simulink model "WECBench"  (R2025b)
settings: Solver=FixedStepAuto  StartTime=0.0  StopTime=inf  RelTol=1e-3
values from neighbouring files (symbols this model uses):
  CL = 13    [initWECBench.m]
  Damping = ExcelGains(:,2)    [initWECBench.m]
  driveKt = 23.6    [initWECBench.m]
  DUTKt = 8.51    [initWECBench.m]
  numPeriods = 10    [initWECBench.m]
  rampTime = 20    [initWECBench.m]
  sprocketPitchRadius = 0.0636651    [initWECBench.m]
  Stiffness = ExcelGains(:,1)    [initWECBench.m]
  Ts = 0.001    [initPendulum.m]    (also in initWECBench.m)
  wavePeriod = 6.00    (= 6)    [initWECBench.m]
libraries: slrealtimeethercatlib x38, slrealtimeloglib x13, dspfdesign x4, simulink x3, dspsrcs4 x2, dspsigops x1, slrealtimeptplib x1, slrealtimetgmanagement x1
settings Model: Creator=bbosma  LastModifiedBy=bosmab
settings SolverCC: ConcurrentTasks=on  PositivePriorityOrder=on
settings DataIOCC: ExternalInput=ds  LoadExternalInput=on
settings OptimizationCC: BlockReduction=off  OptimizeBlockIOStorage=off
settings DebuggingCC: TasksWithSamePriorityMsg=none
settings HardwareCC: ProdBitPerLong=64.0  ProdLongLongMode=on  ProdHWDeviceType=Intel->x86-64 (Linux 64)
settings RTWCC: SystemTargetFile=speedgoat.tlc  TemplateMakefile=slrealtime_default_tmf  RTWVerbose=off  Toolchain=Simulink Real-Time Toolchain  BuildConfiguration=Faster Runs  CodeExecutionProfiling=on  TargetLang=C++  Description=Speedgoat Real-Time Target Machine
settings SimulinkRealTimeTargetCC: SLRTFileLogMaxRuns=1.0  ExtModeMaxTrigDuration=10.0  ExtModeStaticAllocSize=1000000.0  ExtModeTransport=0.0  MultiwordLength=2048.0  DynamicStringBufferSize=256.0  PreserveMATLABNamespacesInGeneratedCode=on  SubcomponentCodeInterfacePackaging=Reusable function  MATLABClassNameForMDSCustomization=Simulink.SoftwareTarget.GRTCustomization  InstructionSetFMA=off  LogToMDFFile=off

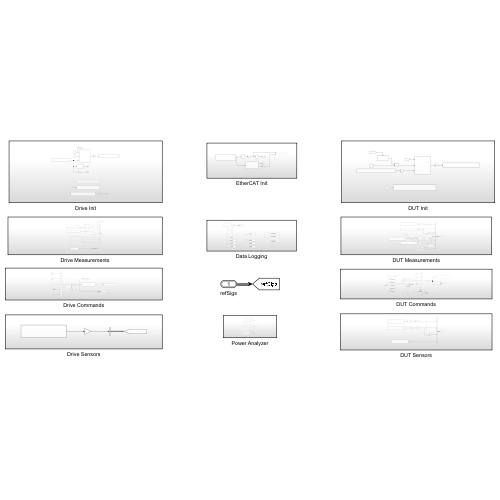
[thumbnail: Simulink's stored preview of the top-level diagram]
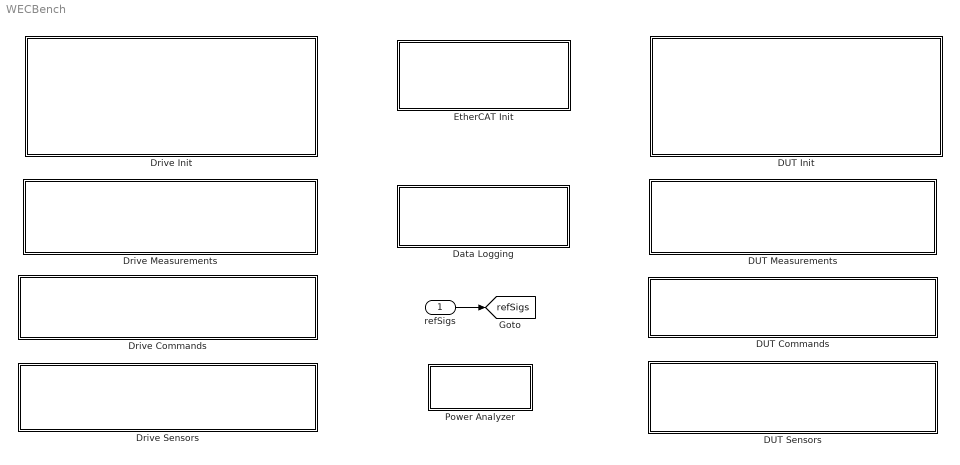
== system WECBench ==
  refSigs : Inport  OutDataTypeStr=Bus: refSigs
  DUT Commands : Subsystem
  DUT Init : Subsystem
  DUT Measurements : Subsystem
  DUT Sensors : Subsystem
  Data Logging : Subsystem
  Drive Commands : Subsystem
  Drive Init : Subsystem
  Drive Measurements : Subsystem
  Drive Sensors : Subsystem
  EtherCAT Init : Subsystem
  Power Analyzer : Subsystem
  tag scope: refSigs=global
  wires:
  refSigs/1 -> [refSigs]

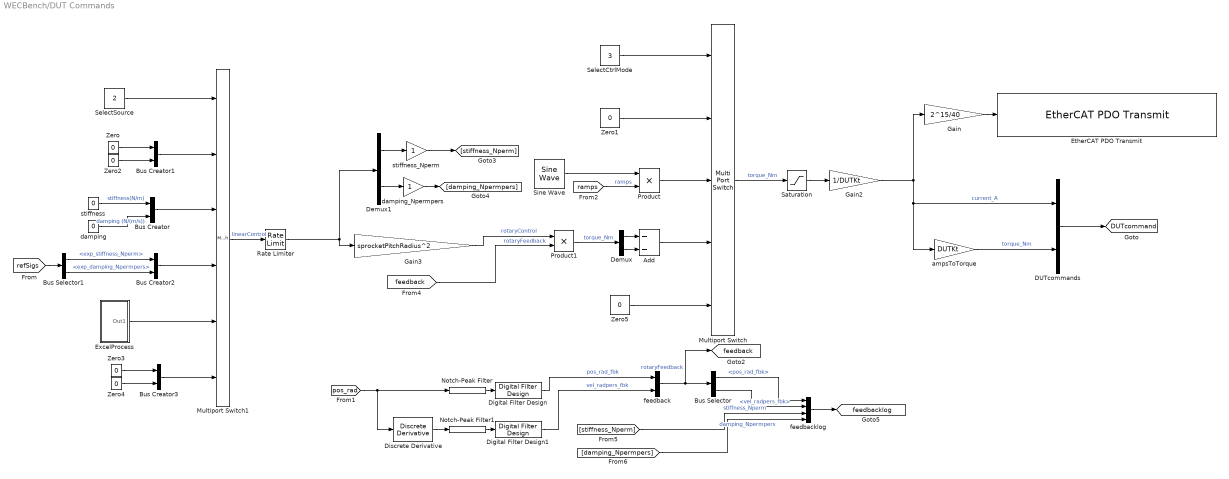
== system WECBench/DUT Commands ==
  Add : Sum  Inputs=--
  Bus Creator{,1..3} (4 alike) : BusCreator  Inputs=2
  Bus Selector : BusSelector  OutputSignals=pos_rad_fbk,vel_radpers_fbk
  Bus Selector1 : BusSelector  OutputSignals=exp_stiffness_Nperm,exp_damping_Npermpers
  DUTcommands : BusCreator  Inputs=2
  Demux : Demux  Outputs=2
  Demux1 : Demux  Outputs=2
  Digital Filter Design : dspfdesign/Digital Filter Design  mwdsp_browser_bugfix_var=off
  Digital Filter Design1 : dspfdesign/Digital Filter Design  mwdsp_browser_bugfix_var=off
  Discrete Derivative : simulink/Discrete/Discrete Derivative  gainval=1.0  ICPrevScaledInput=0.0  OutMin=[]  OutMax=[]  OutDataType=fixdt(1, 16)  OutScaling=2^-10  DoSatur=off
  EtherCAT PDO Transmit : slrealtimeethercatlib/EtherCAT PDO Transmit  Priority=3  sig_name=Drive 7 (AMC - DPE X2.1).PDO data to Slave.Target Current  sig_offset=656  sig_type=int16  type_size=16  sig_dim=1  device_id=0  sample_time=0.001000
  ExcelProcess : Subsystem
  Gain : Gain  Gain=2^15/40  OutDataTypeStr=int16
  Gain2 : Gain  Gain=1/DUTKt
  Gain3 : Gain  Gain=sprocketPitchRadius^2
  Multiport Switch : MultiPortSwitch  DataPortForDefault=Additional data port  SaturateOnIntegerOverflow=off  InputSameDT=off
  Multiport Switch1 : MultiPortSwitch  Inputs=4  DataPortForDefault=Additional data port  SaturateOnIntegerOverflow=off  InputSameDT=off
  Notch-Peak Filter : dspfdesign/Notch-Peak Filter  Specification=Bandwidth and center frequency  BandwidthPort=off  Bandwidth=10  QualityFactorPort=off  QualityFactor=5  CenterFrequencyPort=off  CenterFrequency=50  BandwidthCoefficientPort=off  BandwidthCoefficient=0.72654  CenterFrequencyCoefficientPort=off  CenterFrequencyCoefficient=0  Output=Notch  SampleRateMode=Specify on dialog  SampleRate=1/Ts  SimulateUsing=Code generation
  Notch-Peak Filter1 : dspfdesign/Notch-Peak Filter  Specification=Bandwidth and center frequency  BandwidthPort=off  Bandwidth=10  QualityFactorPort=off  QualityFactor=5  CenterFrequencyPort=off  CenterFrequency=50  BandwidthCoefficientPort=off  BandwidthCoefficient=0.72654  CenterFrequencyCoefficientPort=off  CenterFrequencyCoefficient=0  Output=Notch  SampleRateMode=Specify on dialog  SampleRate=1/Ts  SimulateUsing=Code generation
  Product : Product
  Product1 : Product
  Rate Limiter : RateLimiter  RisingSlewLimit=200  FallingSlewLimit=-200  SampleTimeMode=inherited
  Saturation : Saturate
  SelectCtrlMode : Constant  Value=3  OutDataTypeStr=double
  SelectSource : Constant  Value=2  OutDataTypeStr=double
  Sine Wave : dspsrcs4/Sine Wave  Amplitude=0.2*DUTKt  Frequency=1  Phase=0  SampleMode=Discrete  OutComplex=Real  CompMethod=Trigonometric fcn  TableSize=Speed  SampleTime=Ts  SamplesPerFrame=1  ResetState=Restart at time zero  OutputFrames=off  dataType=double  wordLen=16  udDataType=sfix(16)  fracBitsMode=Best precision  numFracBits=15  OutDataTypeStr=double  LastOutDataTypeStr=double
  Zero{,2..4} (4 alike) : Constant  Value=0  OutDataTypeStr=double
  Zero1 : Constant  Value=0  OutDataTypeStr=Inherit: Inherit via back propagation
  Zero5 : Constant  Value=0  OutDataTypeStr=Inherit: Inherit via back propagation
  ampsToTorque : Gain  Gain=DUTKt
  damping : Constant  Value=0  OutDataTypeStr=double
  damping_Npermpers : Gain
  feedback : BusCreator  Inputs=2
  feedbacklog : BusCreator  Inputs=4
  stiffness : Constant  Value=0  OutDataTypeStr=double
  stiffness_Nperm : Gain
  tag scope: DUTcommand=global, feedback=global, feedbacklog=global
  wires:
  Gain2/1 -> Gain/1, ampsToTorque/1, DUTcommands/1  "current_A"
  Gain/1 -> EtherCAT PDO Transmit/1
  ampsToTorque/1 -> DUTcommands/2  "torque_Nm"
  DUTcommands/1 -> [DUTcommand]
  SelectCtrlMode/1 -> Multiport Switch/1
  Zero1/1 -> Multiport Switch/2
  Multiport Switch/1 -> Saturation/1  "torque_Nm"
  [ramps] -> Product/2  "ramps"
  Sine Wave/1 -> Product/1
  Product/1 -> Multiport Switch/3
  Saturation/1 -> Gain2/1
  [pos_rad] -> Notch-Peak Filter/1, Discrete Derivative/1
  Discrete Derivative/1 -> Notch-Peak Filter1/1
  SelectSource/1 -> Multiport Switch1/1
  Digital Filter Design1/1 -> feedback/2  "vel_radpers_fbk"
  Digital Filter Design/1 -> feedback/1  "pos_rad_fbk"
  Bus Creator/1 -> Multiport Switch1/3
  [feedback] -> Product1/2  "rotaryFeedback"
  Multiport Switch1/1 -> Rate Limiter/1  "linearControl"
  Bus Creator1/1 -> Multiport Switch1/2
  Zero/1 -> Bus Creator1/1
  Demux/2 -> Add/2
  Demux/1 -> Add/1
  Add/1 -> Multiport Switch/4
  Zero2/1 -> Bus Creator1/2
  stiffness/1 -> Bus Creator/1  "stiffness(N/m)"
  damping/1 -> Bus Creator/2  "damping (N/(m/s))"
  feedback/1 -> Bus Selector/1, [feedback]  "rotaryFeedback"
  Product1/1 -> Demux/1  "torque_Nm"
  Gain3/1 -> Product1/1  "rotaryControl"
  [stiffness_Nperm] -> feedbacklog/3  "stiffness_Nperm"
  [damping_Npermpers] -> feedbacklog/4  "damping_Npermpers"
  feedbacklog/1 -> [feedbacklog]
  Bus Selector/2 -> feedbacklog/2  "<vel_radpers_fbk>"
  Bus Selector/1 -> feedbacklog/1  "<pos_rad_fbk>"
  Notch-Peak Filter/1 -> Digital Filter Design/1
  Notch-Peak Filter1/1 -> Digital Filter Design1/1
  [refSigs] -> Bus Selector1/1
  Bus Selector1/1 -> Bus Creator2/1  "<exp_stiffness_Nperm>"
  Bus Selector1/2 -> Bus Creator2/2  "<exp_damping_Npermpers>"
  Bus Creator2/1 -> Multiport Switch1/4
  Demux1/1 -> stiffness_Nperm/1
  Demux1/2 -> damping_Npermpers/1
  stiffness_Nperm/1 -> [stiffness_Nperm]
  damping_Npermpers/1 -> [damping_Npermpers]
  Rate Limiter/1 -> Gain3/1, Demux1/1
  Zero4/1 -> Bus Creator3/2
  Zero3/1 -> Bus Creator3/1
  Bus Creator3/1 -> Multiport Switch1/6
  Zero5/1 -> Multiport Switch/5
  ExcelProcess/1(Out1) -> Multiport Switch1/5

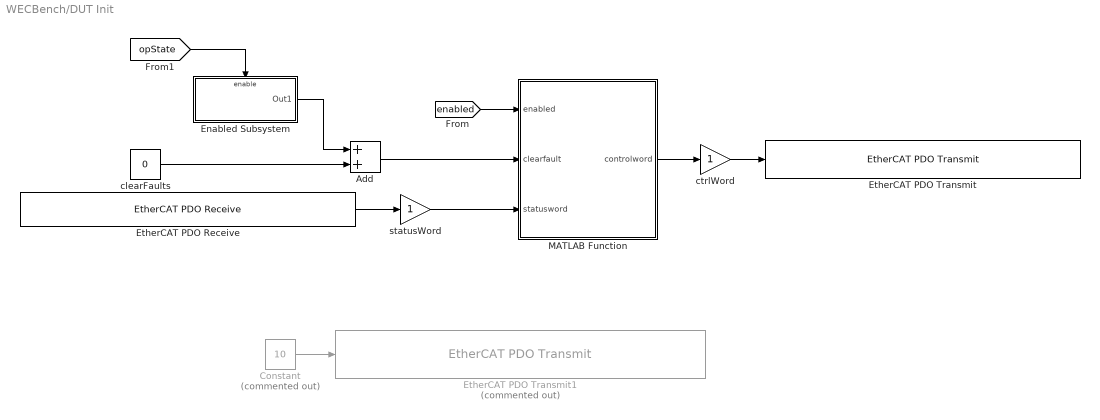
== system WECBench/DUT Init ==
  Add : Sum
  Constant : Constant  Commented=on  Value=10  OutDataTypeStr=int8
  Enabled Subsystem : Subsystem  TreatAsAtomicUnit=on
  EtherCAT PDO Receive : slrealtimeethercatlib/EtherCAT PDO Receive  Priority=2  sig_name=Drive 7 (AMC - DPE X2.1).PDO data from Slave.Status Word  sig_offset=576  sig_type=uint16  type_size=16  sig_dim=1  device_id=0  sample_time=0.001000
  EtherCAT PDO Transmit : slrealtimeethercatlib/EtherCAT PDO Transmit  Priority=3  sig_name=Drive 7 (AMC - DPE X2.1).PDO data to Slave.Control Word  sig_offset=576  sig_type=uint16  type_size=16  sig_dim=1  device_id=0  sample_time=0.001000
  EtherCAT PDO Transmit1 : slrealtimeethercatlib/EtherCAT PDO Transmit  Priority=3  Commented=on  sig_name=Drive 7 (AMC - DPE X2.1).PDO data to Slave.Modes Of Operation  sig_offset=688  sig_type=uint16  type_size=16  sig_dim=1  device_id=0  sample_time=0.001
  MATLAB Function : MATLAB Function  TreatAsAtomicUnit=on
  clearFaults : Constant  Value=0  OutDataTypeStr=Inherit: Inherit via back propagation
  ctrlWord : Gain  OutDataTypeStr=uint16
  statusWord : Gain  OutDataTypeStr=double
  wires:
  ctrlWord/1 -> EtherCAT PDO Transmit/1
  Constant/1 -> EtherCAT PDO Transmit1/1
  MATLAB Function/1(controlword) -> ctrlWord/1
  clearFaults/1 -> Add/2
  EtherCAT PDO Receive/1 -> statusWord/1
  [enabled] -> MATLAB Function/1(enabled)
  statusWord/1 -> MATLAB Function/3(statusword)
  [opState] -> Enabled Subsystem/Enable
  Enabled Subsystem/1(Out1) -> Add/1
  Add/1 -> MATLAB Function/2(clearfault)

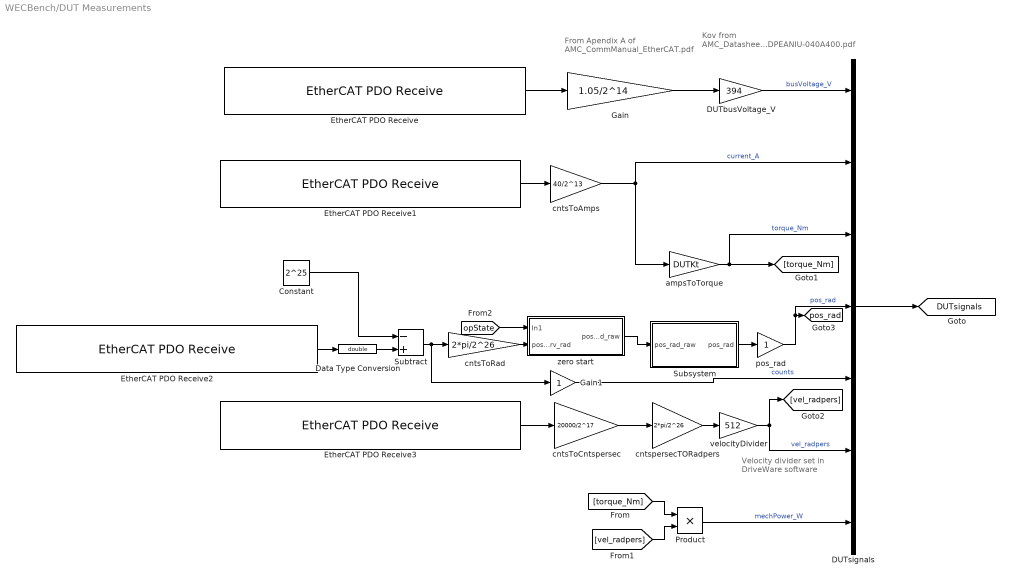
== system WECBench/DUT Measurements ==
  note: Velocity divider set in DriveWare software
  note: Kov from AMC_Datasheet_DPEANIU-040A400.pdf
  note: From Apendix A of AMC_CommManual_EtherCAT.pdf
  Constant : Constant  Value=2^25
  DUTbusVoltage_V : Gain  Gain=394
  DUTsignals : BusCreator  Inputs=7
  Data Type Conversion : DataTypeConversion  OutDataTypeStr=double  SaturateOnIntegerOverflow=off  RndMeth=Floor
  EtherCAT PDO Receive : slrealtimeethercatlib/EtherCAT PDO Receive  Priority=2  sig_name=Drive 7 (AMC - DPE X2.1).PDO data from Slave.DC Bus Voltage  sig_offset=688  sig_type=uint16  type_size=16  sig_dim=1  device_id=0  sample_time=0.001000
  EtherCAT PDO Receive1 : slrealtimeethercatlib/EtherCAT PDO Receive  Priority=2  sig_name=Drive 7 (AMC - DPE X2.1).PDO data from Slave.Actual Current  sig_offset=656  sig_type=int16  type_size=16  sig_dim=1  device_id=0  sample_time=0.001000
  EtherCAT PDO Receive2 : slrealtimeethercatlib/EtherCAT PDO Receive  Priority=2  sig_name=Drive 7 (AMC - DPE X2.1).PDO data from Slave.Actual position  sig_offset=592  sig_type=int32  type_size=32  sig_dim=1  device_id=0  sample_time=0.001000
  EtherCAT PDO Receive3 : slrealtimeethercatlib/EtherCAT PDO Receive  Priority=2  sig_name=Drive 7 (AMC - DPE X2.1).PDO data from Slave.Actual Velocity  sig_offset=624  sig_type=int32  type_size=32  sig_dim=1  device_id=0  sample_time=0.001000
  Gain : Gain  Gain=1.05/2^14  OutDataTypeStr=double
  Gain1 : Gain  OutDataTypeStr=double
  Product : Product
  Subsystem : Subsystem
  Subtract : Sum  Inputs=-+
  ampsToTorque : Gain  Gain=DUTKt
  cntsToAmps : Gain  Gain=40/2^13  OutDataTypeStr=double
  cntsToCntspersec : Gain  Gain=20000/2^17  OutDataTypeStr=double
  cntsToRad : Gain  Gain=2*pi/2^26  OutDataTypeStr=double
  cntspersecTORadpers : Gain  Gain=2*pi/2^26
  pos_rad : Gain
  velocityDivider : Gain  Gain=512
  zero start : Subsystem
  tag scope: DUTsignals=global, pos_rad=global
  wires:
  EtherCAT PDO Receive/1 -> Gain/1
  Gain/1 -> DUTbusVoltage_V/1
  DUTbusVoltage_V/1 -> DUTsignals/1  "busVoltage_V"
  DUTsignals/1 -> [DUTsignals]
  EtherCAT PDO Receive1/1 -> cntsToAmps/1
  cntsToAmps/1 -> ampsToTorque/1, DUTsignals/2  "current_A"
  ampsToTorque/1 -> DUTsignals/3, [torque_Nm]  "torque_Nm"
  Subtract/1 -> Gain1/1, cntsToRad/1
  pos_rad/1 -> [pos_rad], DUTsignals/4  "pos_rad"
  EtherCAT PDO Receive3/1 -> cntsToCntspersec/1
  cntsToCntspersec/1 -> cntspersecTORadpers/1
  cntspersecTORadpers/1 -> velocityDivider/1
  velocityDivider/1 -> [vel_radpers], DUTsignals/6  "vel_radpers"
  [torque_Nm] -> Product/1
  [vel_radpers] -> Product/2
  Product/1 -> DUTsignals/7  "mechPower_W"
  cntsToRad/1 -> zero start/2(pos_drv_rad)
  Subsystem/1(pos_rad) -> pos_rad/1
  Gain1/1 -> DUTsignals/5  "counts"
  EtherCAT PDO Receive2/1 -> Data Type Conversion/1
  Data Type Conversion/1 -> Subtract/2
  Constant/1 -> Subtract/1
  [opState] -> zero start/1(In1)
  zero start/1(pos_rad_raw) -> Subsystem/1(pos_rad_raw)

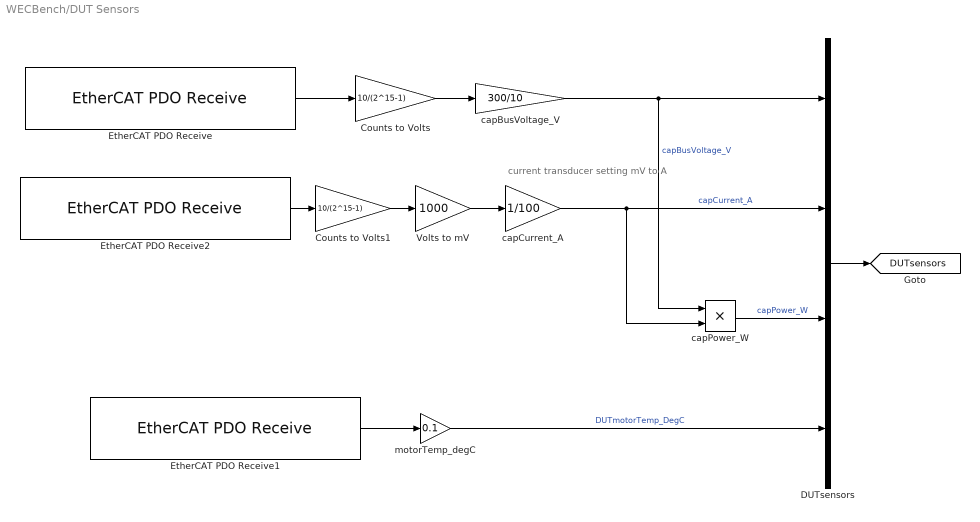
== system WECBench/DUT Sensors ==
  note: current transducer setting mV to A
  Counts to Volts : Gain  Gain=10/(2^15-1)  OutDataTypeStr=double
  Counts to Volts1 : Gain  Gain=10/(2^15-1)  OutDataTypeStr=double
  DUTsensors : BusCreator  Inputs=4
  EtherCAT PDO Receive : slrealtimeethercatlib/EtherCAT PDO Receive  Priority=2  sig_name=Term 13 (EL3104).AI Standard Channel 1.Value  sig_offset=2272  sig_type=int16  type_size=16  sig_dim=1  device_id=0  sample_time=0.001000
  EtherCAT PDO Receive1 : slrealtimeethercatlib/EtherCAT PDO Receive  Priority=2  sig_name=Term 12 (EL3202).RTD Inputs Channel 1.Value  sig_offset=2208  sig_type=int16  type_size=16  sig_dim=1  device_id=0  sample_time=0.001000
  EtherCAT PDO Receive2 : slrealtimeethercatlib/EtherCAT PDO Receive  Priority=2  sig_name=Term 13 (EL3104).AI Standard Channel 2.Value  sig_offset=2304  sig_type=int16  type_size=16  sig_dim=1  device_id=0  sample_time=0.001000
  Volts to mV : Gain  Gain=1000  OutDataTypeStr=double
  capBusVoltage_V : Gain  Gain=300/10
  capCurrent_A : Gain  Gain=1/100  OutDataTypeStr=double
  capPower_W : Product
  motorTemp_degC : Gain  Gain=0.1  OutDataTypeStr=double
  tag scope: DUTsensors=global
  wires:
  EtherCAT PDO Receive/1 -> Counts to Volts/1
  capBusVoltage_V/1 -> capPower_W/1, DUTsensors/1  "capBusVoltage_V"
  DUTsensors/1 -> [DUTsensors]
  Counts to Volts/1 -> capBusVoltage_V/1
  EtherCAT PDO Receive1/1 -> motorTemp_degC/1
  motorTemp_degC/1 -> DUTsensors/4  "DUTmotorTemp_DegC"
  EtherCAT PDO Receive2/1 -> Counts to Volts1/1
  Counts to Volts1/1 -> Volts to mV/1
  Volts to mV/1 -> capCurrent_A/1
  capCurrent_A/1 -> capPower_W/2, DUTsensors/2  "capCurrent_A"
  capPower_W/1 -> DUTsensors/3  "capPower_W"

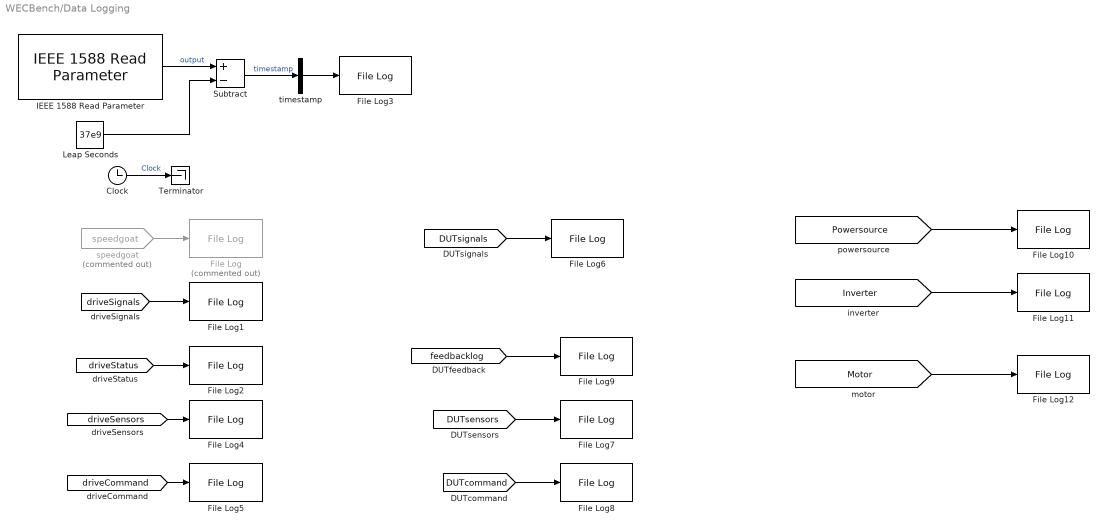
== system WECBench/Data Logging ==
  Clock : Clock
  File Log : slrealtimeloglib/File Log  Commented=on  decimation=1  inputProcessing=Elements as channels (sample based)
  File Log{1..12} (12 alike) : slrealtimeloglib/File Log  decimation=1  inputProcessing=Elements as channels (sample based)
  IEEE 1588 Read Parameter : slrealtimeptplib/IEEE 1588 Read Parameter  Priority=1  ID=1  param=1. System time (nanosecond)  sample_time=Ts
  Leap Seconds : Constant  Value=37e9
  Subtract : Sum  Inputs=+-
  Terminator : Terminator
  speedgoat : From  Commented=on  GotoTag=speedgoat  TagVisibility=global
  timestamp : BusCreator  Inputs=1
  wires:
  speedgoat/1 -> File Log/1
  [driveSignals] -> File Log1/1
  [driveStatus] -> File Log2/1
  Clock/1 -> Terminator/1  "Clock"
  IEEE 1588 Read Parameter/1 -> Subtract/1  "output"
  Leap Seconds/1 -> Subtract/2
  Subtract/1 -> timestamp/1  "timestamp"
  timestamp/1 -> File Log3/1
  [driveSensors] -> File Log4/1
  [driveCommand] -> File Log5/1
  [DUTsignals] -> File Log6/1
  [DUTsensors] -> File Log7/1
  [DUTcommand] -> File Log8/1
  [feedbacklog] -> File Log9/1
  [Powersource] -> File Log10/1
  [Motor] -> File Log12/1
  [Inverter] -> File Log11/1

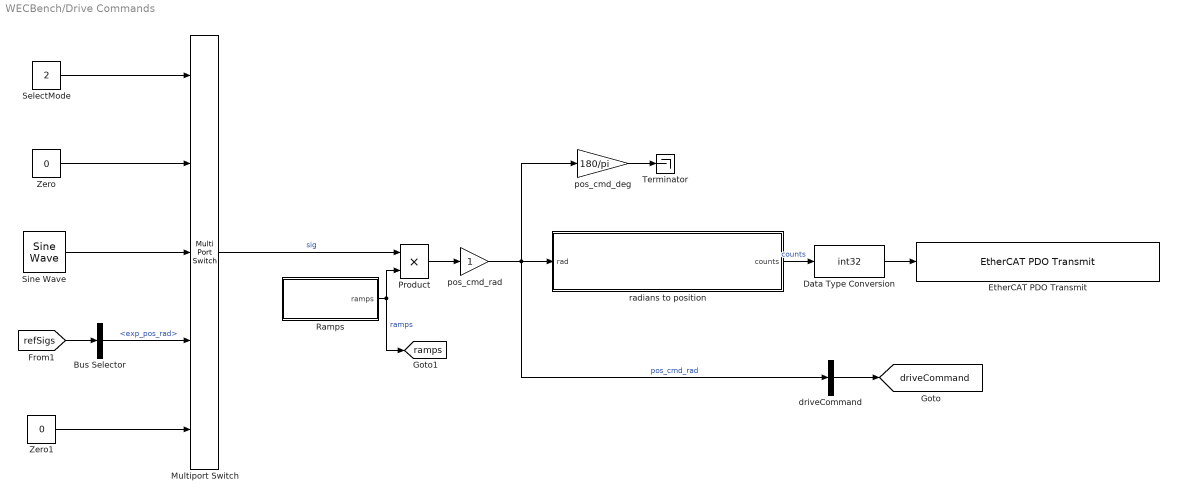
== system WECBench/Drive Commands ==
  Bus Selector : BusSelector  OutputSignals=exp_pos_rad
  Data Type Conversion : DataTypeConversion  OutDataTypeStr=int32  SaturateOnIntegerOverflow=off  RndMeth=Floor
  EtherCAT PDO Transmit : slrealtimeethercatlib/EtherCAT PDO Transmit  Priority=3  sig_name=Drive 4 (Elmo Drive ).Outputs.Target Position  sig_offset=2480  sig_type=int32  type_size=32  sig_dim=1  device_id=0  sample_time=0.001000
  Multiport Switch : MultiPortSwitch  DataPortForDefault=Additional data port  SaturateOnIntegerOverflow=off  InputSameDT=off
  Product : Product
  Ramps : Subsystem
  SelectMode : Constant  Value=2  OutDataTypeStr=double
  Sine Wave : dspsrcs4/Sine Wave  Amplitude=15*pi/180  Frequency=1/5  Phase=0  SampleMode=Discrete  OutComplex=Real  CompMethod=Trigonometric fcn  TableSize=Speed  SampleTime=Ts  SamplesPerFrame=1  ResetState=Restart at time zero  OutputFrames=off  dataType=double  wordLen=16  udDataType=sfix(16)  fracBitsMode=Best precision  numFracBits=15  OutDataTypeStr=double  LastOutDataTypeStr=double
  Terminator : Terminator
  Zero : Constant  Value=0  OutDataTypeStr=double
  Zero1 : Constant  Value=0  OutDataTypeStr=double
  driveCommand : BusCreator  Inputs=1
  pos_cmd_deg : Gain  Gain=180/pi
  pos_cmd_rad : Gain
  radians to position : Subsystem
  tag scope: driveCommand=global, ramps=global
  wires:
  pos_cmd_deg/1 -> Terminator/1
  radians to position/1(counts) -> Data Type Conversion/1  "counts"
  Product/1 -> pos_cmd_rad/1
  SelectMode/1 -> Multiport Switch/1
  Multiport Switch/1 -> Product/1  "sig"
  Ramps/1(ramps) -> [ramps], Product/2  "ramps"
  [refSigs] -> Bus Selector/1
  Bus Selector/1 -> Multiport Switch/4  "<exp_pos_rad>"
  driveCommand/1 -> [driveCommand]
  Sine Wave/1 -> Multiport Switch/3
  Zero/1 -> Multiport Switch/2
  Data Type Conversion/1 -> EtherCAT PDO Transmit/1
  pos_cmd_rad/1 -> radians to position/1(rad), pos_cmd_deg/1, driveCommand/1  "pos_cmd_rad"
  Zero1/1 -> Multiport Switch/5

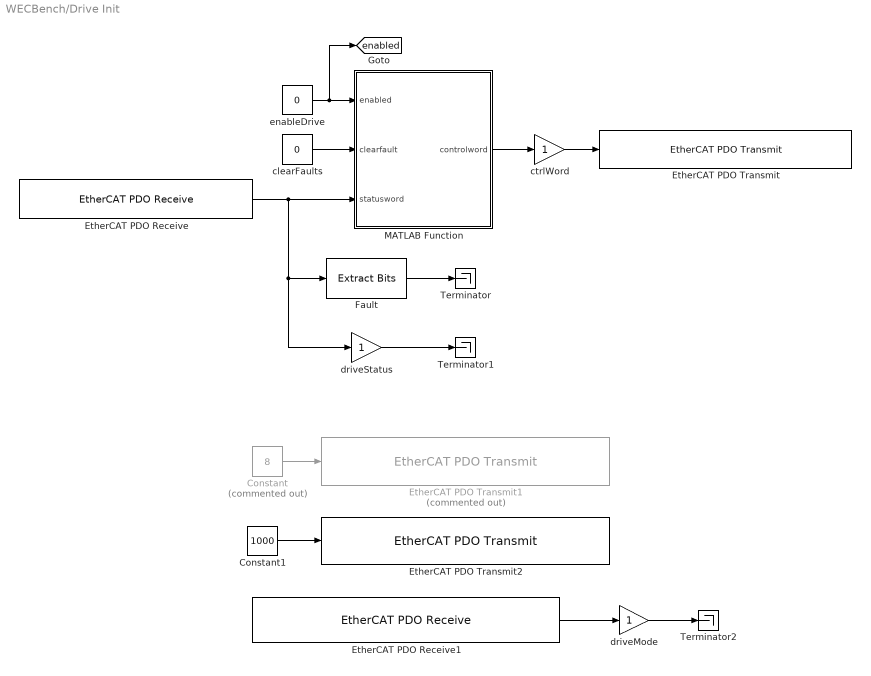
== system WECBench/Drive Init ==
  Constant : Constant  Commented=on  Value=8  OutDataTypeStr=int8
  Constant1 : Constant  Value=1000  OutDataTypeStr=uint16
  EtherCAT PDO Receive : slrealtimeethercatlib/EtherCAT PDO Receive  Priority=2  sig_name=Drive 4 (Elmo Drive ).Inputs.Status word  sig_offset=2480  sig_type=uint16  type_size=16  sig_dim=1  device_id=0  sample_time=0.001000
  EtherCAT PDO Receive1 : slrealtimeethercatlib/EtherCAT PDO Receive  Priority=2  sig_name=Drive 4 (Elmo Drive ).Inputs_1.Mode of operation display  sig_offset=2496  sig_type=int8  type_size=8  sig_dim=1  device_id=0  sample_time=0.001000
  EtherCAT PDO Transmit : slrealtimeethercatlib/EtherCAT PDO Transmit  Priority=3  sig_name=Drive 4 (Elmo Drive ).Outputs.Control word  sig_offset=2560  sig_type=uint16  type_size=16  sig_dim=1  device_id=0  sample_time=0.001000
  EtherCAT PDO Transmit1 : slrealtimeethercatlib/EtherCAT PDO Transmit  Priority=3  Commented=on  sig_name=Uninitialized Block  sig_offset=1  sig_type=boolean  type_size=1  sig_dim=1  device_id=0  sample_time=1
  EtherCAT PDO Transmit2 : slrealtimeethercatlib/EtherCAT PDO Transmit  Priority=3  sig_name=Drive 4 (Elmo Drive ).Outputs.Max. Torque  sig_offset=2544  sig_type=uint16  type_size=16  sig_dim=1  device_id=0  sample_time=0.001000
  Fault : simulink/Logic and Bit Operations/Extract Bits  bitsToExtract=Range of bits  numBits=8  bitIdxRange=[3]  outScalingMode=Preserve fixed-point scaling
  MATLAB Function : MATLAB Function  TreatAsAtomicUnit=on
  Terminator : Terminator
  Terminator1 : Terminator
  Terminator2 : Terminator
  clearFaults : Constant  Value=0  OutDataTypeStr=Inherit: Inherit via back propagation
  ctrlWord : Gain  OutDataTypeStr=uint16
  driveMode : Gain  OutDataTypeStr=double
  driveStatus : Gain  OutDataTypeStr=double
  enableDrive : Constant  Value=0  OutDataTypeStr=double
  tag scope: enabled=global
  wires:
  EtherCAT PDO Receive/1 -> driveStatus/1, Fault/1, MATLAB Function/3(statusword)
  EtherCAT PDO Receive1/1 -> driveMode/1
  clearFaults/1 -> MATLAB Function/2(clearfault)
  MATLAB Function/1(controlword) -> ctrlWord/1
  Constant/1 -> EtherCAT PDO Transmit1/1
  Fault/1 -> Terminator/1
  driveMode/1 -> Terminator2/1
  ctrlWord/1 -> EtherCAT PDO Transmit/1
  driveStatus/1 -> Terminator1/1
  enableDrive/1 -> [enabled], MATLAB Function/1(enabled)
  Constant1/1 -> EtherCAT PDO Transmit2/1

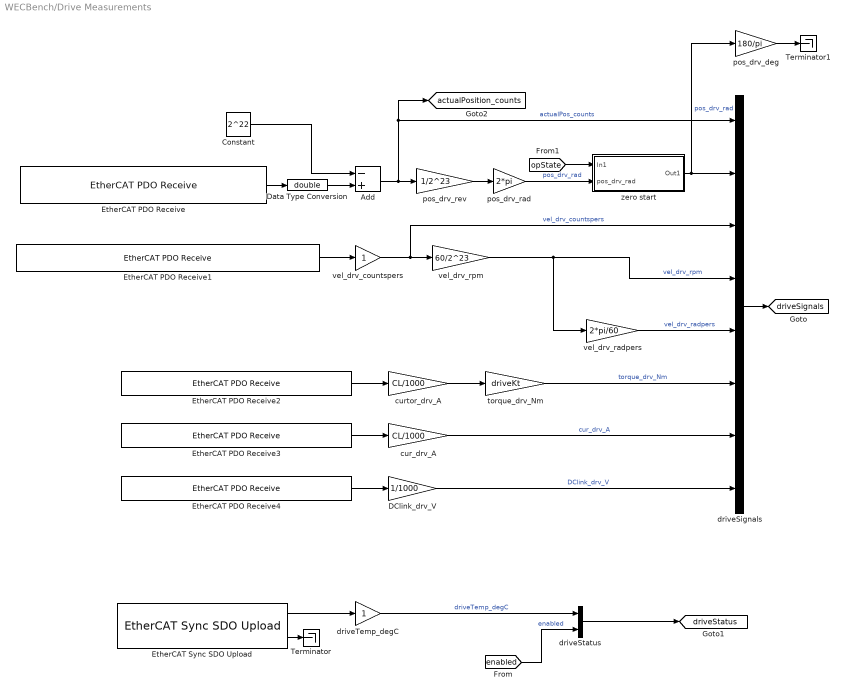
== system WECBench/Drive Measurements ==
  Add : Sum  Inputs=-+
  Constant : Constant  Value=2^22
  DClink_drv_V : Gain  Gain=1/1000  OutDataTypeStr=double
  Data Type Conversion : DataTypeConversion  OutDataTypeStr=double  SaturateOnIntegerOverflow=off  RndMeth=Floor
  EtherCAT PDO Receive : slrealtimeethercatlib/EtherCAT PDO Receive  Priority=2  sig_name=Drive 4 (Elmo Drive ).Inputs_2.Actual position [counts]  sig_offset=2512  sig_type=int32  type_size=32  sig_dim=1  device_id=0  sample_time=0.001000
  EtherCAT PDO Receive1 : slrealtimeethercatlib/EtherCAT PDO Receive  Priority=2  sig_name=Drive 4 (Elmo Drive ).Inputs_3.Velocity sensor actual value [counts/sec]  sig_offset=2544  sig_type=int32  type_size=32  sig_dim=1  device_id=0  sample_time=0.001000
  EtherCAT PDO Receive2 : slrealtimeethercatlib/EtherCAT PDO Receive  Priority=2  sig_name=Drive 4 (Elmo Drive ).Inputs_4.Torque actual value  sig_offset=2576  sig_type=int16  type_size=16  sig_dim=1  device_id=0  sample_time=0.001000
  EtherCAT PDO Receive3 : slrealtimeethercatlib/EtherCAT PDO Receive  Priority=2  sig_name=Drive 4 (Elmo Drive ).Inputs_6.Current actual value  sig_offset=2624  sig_type=int16  type_size=16  sig_dim=1  device_id=0  sample_time=0.001000
  EtherCAT PDO Receive4 : slrealtimeethercatlib/EtherCAT PDO Receive  Priority=2  sig_name=Drive 4 (Elmo Drive ).Inputs_5.DC link circuit voltage  sig_offset=2592  sig_type=uint32  type_size=32  sig_dim=1  device_id=0  sample_time=0.001000
  EtherCAT Sync SDO Upload : slrealtimeethercatlib/EtherCAT Sync SDO Upload  index=0x22A3  subIndex=1  sig_type=int16  sig_dim=1  device_id=0  subdevice_name=Drive 4 (Elmo Drive )  sample_time=1  subdevice_addr=1004  selected_subdevice=Term 1 (EK1100)  timeout=500  subdevice_found=1  complete=0
  Terminator : Terminator
  Terminator1 : Terminator
  cur_drv_A : Gain  Gain=CL/1000  OutDataTypeStr=double
  curtor_drv_A : Gain  Gain=CL/1000  OutDataTypeStr=double
  driveSignals : BusCreator  Inputs=8
  driveStatus : BusCreator  Inputs=2
  driveTemp_degC : Gain  OutDataTypeStr=double
  pos_drv_deg : Gain  Gain=180/pi
  pos_drv_rad : Gain  Gain=2*pi
  pos_drv_rev : Gain  Gain=1/2^23
  torque_drv_Nm : Gain  Gain=driveKt
  vel_drv_countspers : Gain  OutDataTypeStr=double
  vel_drv_radpers : Gain  Gain=2*pi/60
  vel_drv_rpm : Gain  Gain=60/2^23
  zero start : Subsystem
  tag scope: actualPosition_counts=global, driveSignals=global, driveStatus=global
  wires:
  Add/1 -> driveSignals/1, [actualPosition_counts], pos_drv_rev/1  "actualPos_counts"
  pos_drv_rev/1 -> pos_drv_rad/1
  pos_drv_rad/1 -> zero start/2(pos_drv_rad)  "pos_drv_rad"
  EtherCAT PDO Receive/1 -> Data Type Conversion/1
  driveSignals/1 -> [driveSignals]
  EtherCAT PDO Receive1/1 -> vel_drv_countspers/1
  vel_drv_countspers/1 -> vel_drv_rpm/1, driveSignals/3  "vel_drv_countspers"
  vel_drv_rpm/1 -> driveSignals/4, vel_drv_radpers/1  "vel_drv_rpm"
  vel_drv_radpers/1 -> driveSignals/5  "vel_drv_radpers"
  EtherCAT PDO Receive2/1 -> curtor_drv_A/1
  curtor_drv_A/1 -> torque_drv_Nm/1
  torque_drv_Nm/1 -> driveSignals/6  "torque_drv_Nm"
  EtherCAT PDO Receive3/1 -> cur_drv_A/1
  cur_drv_A/1 -> driveSignals/7  "cur_drv_A"
  EtherCAT PDO Receive4/1 -> DClink_drv_V/1
  DClink_drv_V/1 -> driveSignals/8  "DClink_drv_V"
  EtherCAT Sync SDO Upload/1 -> driveTemp_degC/1
  driveTemp_degC/1 -> driveStatus/1  "driveTemp_degC"
  driveStatus/1 -> [driveStatus]
  EtherCAT Sync SDO Upload/2 -> Terminator/1
  pos_drv_deg/1 -> Terminator1/1
  [enabled] -> driveStatus/2  "enabled"
  Data Type Conversion/1 -> Add/2
  Constant/1 -> Add/1
  [opState] -> zero start/1(In1)
  zero start/1(Out1) -> pos_drv_deg/1, driveSignals/2  "pos_drv_rad"

== system WECBench/Drive Sensors ==
  EtherCAT PDO Receive : slrealtimeethercatlib/EtherCAT PDO Receive  Priority=2  sig_name=Term 2 (EL3201).RTD.Value  sig_offset=1696  sig_type=int16  type_size=16  sig_dim=1  device_id=0  sample_time=0.001000
  driveSensors : BusCreator  Inputs=1
  motorTemp_degC : Gain  Gain=0.1  OutDataTypeStr=double
  tag scope: driveSensors=global
  wires:
  EtherCAT PDO Receive/1 -> motorTemp_degC/1
  motorTemp_degC/1 -> driveSensors/1  "motorTemp_degC"
  driveSensors/1 -> [driveSensors]

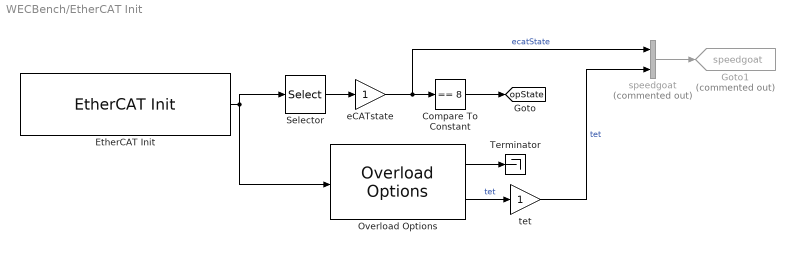
== system WECBench/EtherCAT Init ==
  Compare To Constant : simulink/Logic and Bit Operations/Compare To Constant  relop===  const=8  OutDataTypeStr=boolean
  EtherCAT Init : slrealtimeethercatlib/EtherCAT Init  Priority=0  config_file=C:\Software\WEC-Bench\Simulink\EtherCAT\DriveAndDUTAndPAXML.xml  device_id=0  portnum=1  initstate=2  dctuning=0  enaDebug=0  logFile='c:\dbglog.txt'  sample_time=0.001000  DCMode=2
  Goto1 : Goto  Commented=on  GotoTag=speedgoat  TagVisibility=global
  Overload Options : slrealtimetgmanagement/Overload Options  startupDur=1  startupDurSrc=Tunable Parameter  maxOverload=0  maxOverloadSrc=Tunable Parameter  TETFlag=on
  Selector : Selector  InputPortWidth=6  IndexOptions=Index vector (dialog)  Indices=[2]  OutputSizes=1
  Terminator : Terminator
  eCATstate : Gain  OutDataTypeStr=double
  speedgoat : BusCreator  Commented=on  Inputs=2
  tet : Gain  OutDataTypeStr=double
  tag scope: opState=global
  wires:
  speedgoat/1 -> Goto1/1
  eCATstate/1 -> speedgoat/1, Compare To Constant/1  "ecatState"
  EtherCAT Init/1 -> Overload Options/1, Selector/1
  Overload Options/2 -> tet/1  "tet"
  tet/1 -> speedgoat/2  "tet"
  Selector/1 -> eCATstate/1
  Compare To Constant/1 -> [opState]
  Overload Options/1 -> Terminator/1

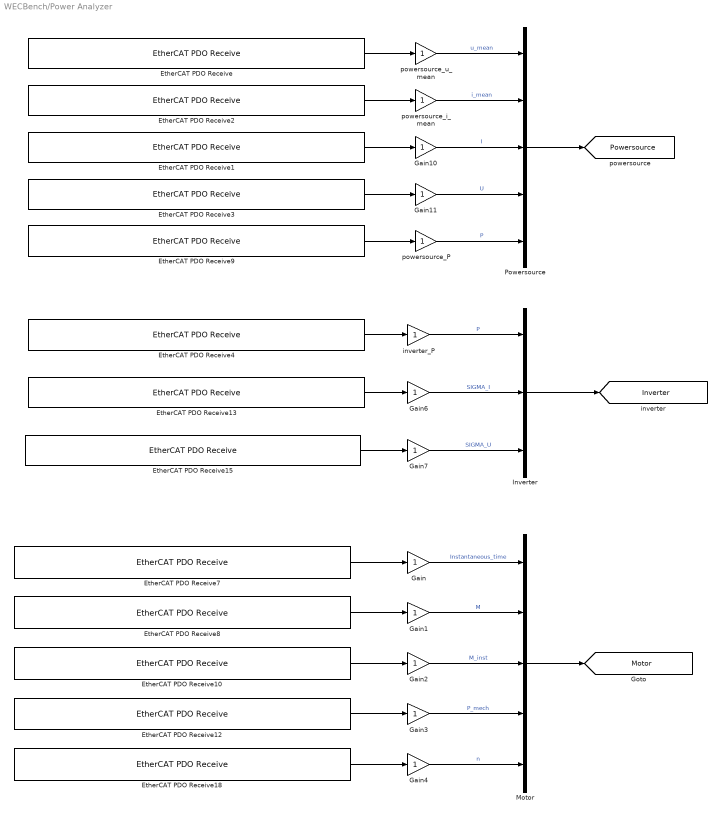
== system WECBench/Power Analyzer ==
  EtherCAT PDO Receive : slrealtimeethercatlib/EtherCAT PDO Receive  Priority=2  sig_name=Box 30 (GEN Series DAQ System).Powersource.out.u_mean.Powersource.out.u_mean_V  sig_offset=944  sig_type=single  type_size=32  sig_dim=1  device_id=0  sample_time=0.001000
  EtherCAT PDO Receive1 : slrealtimeethercatlib/EtherCAT PDO Receive  Priority=2  sig_name=Box 30 (GEN Series DAQ System).Powersource.out.I.Powersource.out.I_V  sig_offset=824  sig_type=single  type_size=32  sig_dim=1  device_id=0  sample_time=0.001000
  EtherCAT PDO Receive10 : slrealtimeethercatlib/EtherCAT PDO Receive  Priority=2  sig_name=Box 30 (GEN Series DAQ System).Motor.out.M_inst.Motor.out.M_inst_V  sig_offset=1144  sig_type=single  type_size=32  sig_dim=1  device_id=0  sample_time=0.001000
  EtherCAT PDO Receive12 : slrealtimeethercatlib/EtherCAT PDO Receive  Priority=2  sig_name=Box 30 (GEN Series DAQ System).Motor.out.P_mech.Motor.out.P_mech_V  sig_offset=1224  sig_type=single  type_size=32  sig_dim=1  device_id=0  sample_time=0.001000
  EtherCAT PDO Receive13 : slrealtimeethercatlib/EtherCAT PDO Receive  Priority=2  sig_name=Box 30 (GEN Series DAQ System).Inverter.out.SIGMA_I.Inverter.out.SIGMA_I_V  sig_offset=1304  sig_type=single  type_size=32  sig_dim=1  device_id=0  sample_time=0.001000
  EtherCAT PDO Receive15 : slrealtimeethercatlib/EtherCAT PDO Receive  Priority=2  sig_name=Box 30 (GEN Series DAQ System).Inverter.out.SIGMA_U.Inverter.out.SIGMA_U_V  sig_offset=1344  sig_type=single  type_size=32  sig_dim=1  device_id=0  sample_time=0.001000
  EtherCAT PDO Receive18 : slrealtimeethercatlib/EtherCAT PDO Receive  Priority=2  sig_name=Box 30 (GEN Series DAQ System).Motor.out.n.Motor.out.n_V  sig_offset=1104  sig_type=single  type_size=32  sig_dim=1  device_id=0  sample_time=0.001000
  EtherCAT PDO Receive2 : slrealtimeethercatlib/EtherCAT PDO Receive  Priority=2  sig_name=Box 30 (GEN Series DAQ System).Powersource.out.i_mean.Powersource.out.i_mean_V  sig_offset=904  sig_type=single  type_size=32  sig_dim=1  device_id=0  sample_time=0.001000
  EtherCAT PDO Receive3 : slrealtimeethercatlib/EtherCAT PDO Receive  Priority=2  sig_name=Box 30 (GEN Series DAQ System).Powersource.out.U.Powersource.out.U_V  sig_offset=864  sig_type=single  type_size=32  sig_dim=1  device_id=0  sample_time=0.001000
  EtherCAT PDO Receive4 : slrealtimeethercatlib/EtherCAT PDO Receive  Priority=2  sig_name=Box 30 (GEN Series DAQ System).Inverter.out.P.Inverter.out.P_V  sig_offset=1024  sig_type=single  type_size=32  sig_dim=1  device_id=0  sample_time=0.001000
  EtherCAT PDO Receive7 : slrealtimeethercatlib/EtherCAT PDO Receive  Priority=2  sig_name=Box 30 (GEN Series DAQ System).Motor.out.Instantaneous_time.Motor.out.Instantaneous_time_V  sig_offset=1264  sig_type=single  type_size=32  sig_dim=1  device_id=0  sample_time=0.001000
  EtherCAT PDO Receive8 : slrealtimeethercatlib/EtherCAT PDO Receive  Priority=2  sig_name=Box 30 (GEN Series DAQ System).Motor.out.M.Motor.out.M_V  sig_offset=1064  sig_type=single  type_size=32  sig_dim=1  device_id=0  sample_time=0.001000
  EtherCAT PDO Receive9 : slrealtimeethercatlib/EtherCAT PDO Receive  Priority=2  sig_name=Box 30 (GEN Series DAQ System).Powersource.out.P.Powersource.out.P_V  sig_offset=984  sig_type=single  type_size=32  sig_dim=1  device_id=0  sample_time=0.001000
  Gain{,1..4,6..7,10..11} (9 alike) : Gain  OutDataTypeStr=double
  Inverter : BusCreator  Inputs=3
  Motor : BusCreator  Inputs=5
  Powersource : BusCreator  Inputs=5
  inverter_P : Gain  OutDataTypeStr=double
  powersource_P : Gain  OutDataTypeStr=double
  powersource_i_mean : Gain  OutDataTypeStr=double
  powersource_u_mean : Gain  OutDataTypeStr=double
  tag scope: Inverter=global, Motor=global, Powersource=global
  wires:
  powersource_u_mean/1 -> Powersource/1  "u_mean"
  powersource_i_mean/1 -> Powersource/2  "i_mean"
  inverter_P/1 -> Inverter/1  "P"
  Gain6/1 -> Inverter/2  "SIGMA_I"
  Gain7/1 -> Inverter/3  "SIGMA_U"
  Gain/1 -> Motor/1  "Instantaneous_time"
  Gain1/1 -> Motor/2  "M"
  Gain2/1 -> Motor/3  "M_inst"
  Gain3/1 -> Motor/4  "P_mech"
  Gain4/1 -> Motor/5  "n"
  Powersource/1 -> [Powersource]
  Inverter/1 -> [Inverter]
  Motor/1 -> [Motor]
  EtherCAT PDO Receive7/1 -> Gain/1
  EtherCAT PDO Receive8/1 -> Gain1/1
  EtherCAT PDO Receive10/1 -> Gain2/1
  EtherCAT PDO Receive12/1 -> Gain3/1
  EtherCAT PDO Receive18/1 -> Gain4/1
  Gain10/1 -> Powersource/3  "I"
  Gain11/1 -> Powersource/4  "U"
  EtherCAT PDO Receive4/1 -> inverter_P/1
  EtherCAT PDO Receive13/1 -> Gain6/1
  EtherCAT PDO Receive15/1 -> Gain7/1
  EtherCAT PDO Receive/1 -> powersource_u_mean/1
  EtherCAT PDO Receive2/1 -> powersource_i_mean/1
  EtherCAT PDO Receive1/1 -> Gain10/1
  EtherCAT PDO Receive3/1 -> Gain11/1
  EtherCAT PDO Receive9/1 -> powersource_P/1
  powersource_P/1 -> Powersource/5  "P"

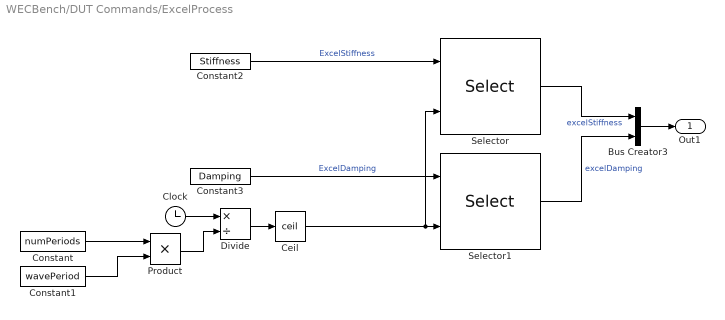
== system WECBench/DUT Commands/ExcelProcess ==
  Bus Creator3 : BusCreator  Inputs=2
  Ceil : Rounding  Operator=ceil
  Clock : Clock
  Constant : Constant  Value=numPeriods
  Constant1 : Constant  Value=wavePeriod
  Constant2 : Constant  Value=Stiffness  OutDataTypeStr=double
  Constant3 : Constant  Value=Damping  OutDataTypeStr=double
  Divide : Product  Inputs=*/
  Product : Product
  Selector : Selector  InputPortWidth=ExcelLength  IndexOptions=Index vector (port)  Indices=[1 3]  OutputSizes=1
  Selector1 : Selector  InputPortWidth=ExcelLength  IndexOptions=Index vector (port)  Indices=[1 3]  OutputSizes=1
  Out1 : Outport
  wires:
  Bus Creator3/1 -> Out1/1
  Selector/1 -> Bus Creator3/1  "excelStiffness"
  Divide/1 -> Ceil/1
  Clock/1 -> Divide/1
  Product/1 -> Divide/2
  Ceil/1 -> Selector/2, Selector1/2
  Constant2/1 -> Selector/1  "ExcelStiffness"
  Constant3/1 -> Selector1/1  "ExcelDamping"
  Selector1/1 -> Bus Creator3/2  "excelDamping"
  Constant/1 -> Product/1
  Constant1/1 -> Product/2

== system WECBench/DUT Init/Enabled Subsystem ==
  Enable : EnablePort
  Delay : Delay  DelayLength=1/Ts
  One : Constant  OutDataTypeStr=Inherit: Inherit via back propagation
  One1 : Constant  Value=-1  OutDataTypeStr=Inherit: Inherit via back propagation
  Sum : Sum  Inputs=|++
  Out1 : Outport
  wires:
  Sum/1 -> Out1/1
  One/1 -> Sum/1
  One1/1 -> Delay/1
  Delay/1 -> Sum/2

== system WECBench/DUT Measurements/Subsystem ==
  pos_rad_raw : Inport
  Sample and Hold : dspsigops/Sample and Hold  trig=Rising edge  initCond=0  latchinput=off
  Subtract : Sum  Inputs=-+
  pos_rad : Outport
  wires:
  [EnableRamps] -> Sample and Hold/Trigger
  Sample and Hold/1 -> Subtract/1
  pos_rad_raw/1 -> Sample and Hold/1, Subtract/2
  Subtract/1 -> pos_rad/1

== system WECBench/DUT Measurements/zero start ==
  In1 : Inport
  pos_drv_rad : Inport  Port=2
  Switch : Switch  Criteria=u2 > Threshold  SaturateOnIntegerOverflow=off  InputSameDT=off
  Zero : Constant  Value=0  OutDataTypeStr=double
  pos_rad_raw : Outport
  wires:
  In1/1 -> Switch/2
  Switch/1 -> pos_rad_raw/1
  pos_drv_rad/1 -> Switch/1
  Zero/1 -> Switch/3

== system WECBench/Drive Commands/Ramps ==
  EnableRamps : Constant  Value=0  OutDataTypeStr=double
  Rate Limiter : RateLimiter  RisingSlewLimit=1/rampTime  FallingSlewLimit=-1/rampTime  SampleTimeMode=inherited
  ramps : Outport
  tag scope: EnableRamps=global
  wires:
  EnableRamps/1 -> [EnableRamps], Rate Limiter/1
  Rate Limiter/1 -> ramps/1

== system WECBench/Drive Commands/radians to position ==
  rad : Inport
  Constant : Constant  Value=2^22
  Delay : Delay  DelayLength=1*1000  InputProcessing=Columns as channels (frame based)
  Rate Limiter : RateLimiter  RisingSlewLimit=1e6  FallingSlewLimit=-1e6  SampleTimeMode=inherited
  Subtract : Sum
  Switch : Switch  Criteria=u2 > Threshold  SaturateOnIntegerOverflow=off  InputSameDT=off
  Zero : Constant  Value=0  OutDataTypeStr=double
  radtocounts : Gain  Gain=2^23/(2*pi)
  counts : Outport
  wires:
  [enabled] -> Delay/1
  rad/1 -> radtocounts/1
  Delay/1 -> Switch/2
  Zero/1 -> Switch/3
  Switch/1 -> Rate Limiter/1
  Rate Limiter/1 -> Subtract/2
  radtocounts/1 -> Switch/1
  Subtract/1 -> counts/1
  Constant/1 -> Subtract/1

== system WECBench/Drive Measurements/zero start ==
  In1 : Inport
  pos_drv_rad : Inport  Port=2
  Switch : Switch  Criteria=u2 > Threshold  SaturateOnIntegerOverflow=off  InputSameDT=off
  Zero : Constant  Value=0  OutDataTypeStr=double
  Out1 : Outport
  wires:
  In1/1 -> Switch/2
  Switch/1 -> Out1/1
  pos_drv_rad/1 -> Switch/1
  Zero/1 -> Switch/3

== matlab function WECBench/Drive Init/MATLAB Function ==
  data: enabled input; controlword output; clearfault input; statusword input
function controlword = fcn(enabled, clearfault, statusword)

bitstatus = bitget(statusword,1:16);

if ~clearfault
    if enabled
        if bitstatus(1) == 0 % Ready to switch on not ready
            controlword = 6; % command ready switch on
        elseif ~bitstatus(2) % switched not yet on
            controlword = 7; % command switch on
        elseif ~bitstatus(3) % operation not yet enabled
            controlword = 15; % command enable
        else
            controlword = 15; % maintain enabled state
        end
    else
        controlword = 4; % command disabled
    end
else
    controlword = 128; % command clear faults
end

== matlab function WECBench/DUT Init/MATLAB Function ==
  data: enabled input; controlword output; clearfault input; statusword input
function controlword = fcn(enabled, clearfault, statusword)

bitstatus = bitget(statusword,1:16);

if ~clearfault
    if enabled
        if bitstatus(1) == 0 % Ready to switch on not ready
            controlword = 6; % command ready switch on
        elseif ~bitstatus(2) % switched not yet on
            controlword = 7; % command switch on
        elseif ~bitstatus(3) % operation not yet enabled
            controlword = 15; % command enable
        else
            controlword = 15; % maintain enabled state
        end
    else
        controlword = 4; % command disabled
    end
else
    controlword = 128; % command clear faults
end
